simulink model "frequencycount"  (Simulink 10.1)
settings: Solver=ode45  StartTime=0.0  StopTime=2.5  FixedStep=5e-6  RelTol=1e-4  EnableMultiTasking=on
libraries: simulink x1
settings Model: Creator=mf  LastModifiedBy=Lukas Bilal  ExtModeAutoUpdateStatusClock=off
settings DataIOCC: LimitDataPoints=on  SignalLoggingSaveFormat=ModelDataLogs  SignalLoggingName=sigsOut
settings OptimizationCC: BooleanDataType=off  ExpressionDepthLimit=2147483647
settings DebuggingCC: SaveWithParameterizedLinksMsg=none  SignalResolutionControl=TryResolveAllWithWarning  MultiTaskDSMMsg=warning  MultiTaskCondExecSysMsg=none  StateNameClashWarn=warning
settings HardwareCC: TargetUnknown=on
settings SFSimCC: SimParseCustomCode=off

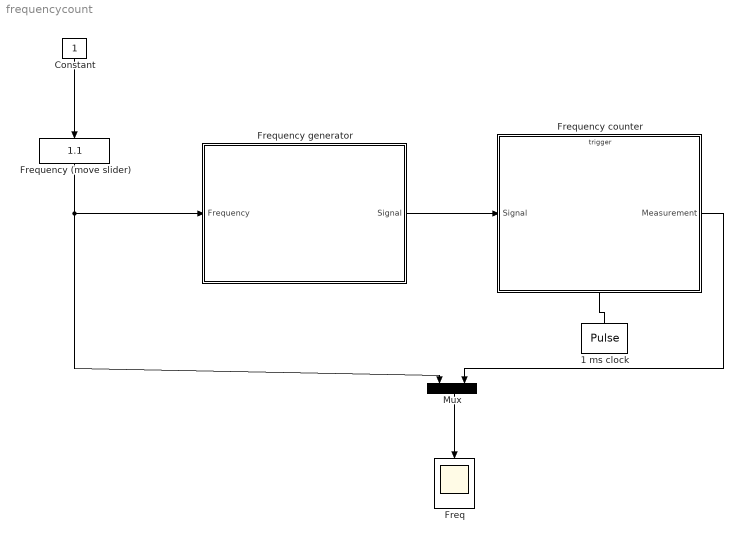
== system frequencycount ==
  1 ms clock : DiscretePulseGenerator  PulseType=Time based  Period=1e-3  PulseWidth=50
  Constant : Constant
  Freq : Scope
  Frequency (move slider) : simulink/Math Operations/Slider Gain  gain=1.1  low=1  high=500
  Frequency counter : Stateflow chart  TreatAsAtomicUnit=on
  Frequency generator : Subsystem
  Mux : Mux  Inputs=2
  wires:
  Constant/1 -> Frequency (move slider)/1
  1 ms clock/1 -> Frequency counter/Trigger
  Mux/1 -> Freq/1
  Frequency (move slider)/1 -> Frequency generator/1(Frequency), Mux/1
  Frequency counter/1(Measurement) -> Mux/2
  Frequency generator/1(Signal) -> Frequency counter/1(Signal)

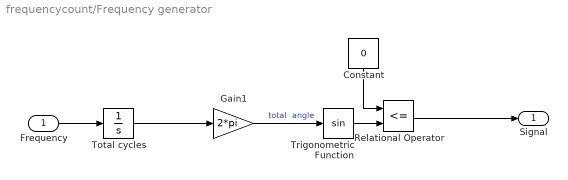
== system frequencycount/Frequency generator ==
  Frequency : Inport
  Constant : Constant  Value=0
  Gain1 : Gain  Gain=2*pi  SaturateOnIntegerOverflow=on  OutDataTypeStr=Inherit: Same as input  ParamDataTypeStr=Inherit: Same as input
  Relational Operator : RelationalOperator  Operator=<=  OutDataTypeStr=boolean  RndMeth=Nearest
  Total cycles : Integrator
  Trigonometric Function : Trigonometry
  Signal : Outport
  wires:
  Frequency/1 -> Total cycles/1
  Trigonometric Function/1 -> Relational Operator/2
  Constant/1 -> Relational Operator/1
  Relational Operator/1 -> Signal/1
  Total cycles/1 -> Gain1/1
  Gain1/1 -> Trigonometric Function/1  "total  angle"

== stateflow chart Frequency counter ==
  settings: executeAtInitialization=1
  state FrequencyCounter
    state Clock [parallel]
      settings: executionOrder=1
      state Clock
      (default) -> FrequencyCounter.Clock.Clock
      FrequencyCounter.Clock.Clock -> FrequencyCounter.Clock.Clock : clk [time < 1000]
          | {
          |   time++;
          | }
    state Counter [parallel]
      settings: executionOrder=2
      state Counter
      FrequencyCounter.Counter.Counter -> FrequencyCounter.Counter.Counter [order 1] : [time == 1000]
          | {
          |   Measurement = counter;
          | }
      FrequencyCounter.Counter.Counter -> FrequencyCounter.Counter.Counter [order 2] : [time < 1000 && Signal && hasChanged(Signal)]
          | {
          |   counter++;
          | }
  (default) -> FrequencyCounter
  data: Measurement output double; time local double =double(0); Signal input boolean; counter local double =double(0)
  events: clk input RISING_EDGE_EVENT
